simulink model "SimulinkElektrotechnikR2020"  (R2021b)
settings: Solver=FixedStepAuto  StartTime=0.0  StopTime=100  FixedStep=0.00001  RelTol=1e-3
undefined symbols (not defined in the file): C, L, R
settings Model: Creator=PM  LastModifiedBy=metzler
settings SolverCC: AlgebraicLoopSolver=TrustRegion
settings DebuggingCC: UnconnectedInputMsg=none  UnconnectedOutputMsg=none  UnconnectedLineMsg=none  SFMachineParentedDataDiag=warning
settings ModelReferenceCC: EnableRefExpFcnMdlSchedulingChecks=off

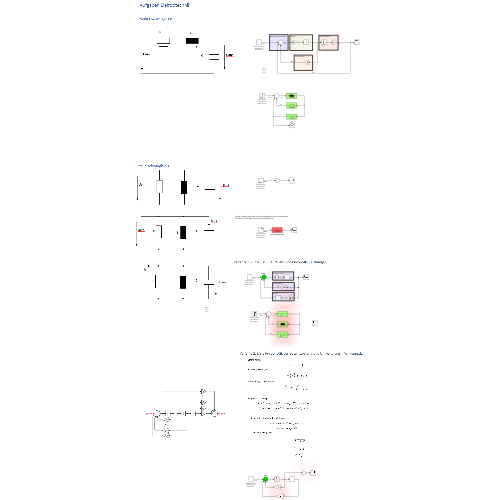
[thumbnail: Simulink's stored preview of the top-level diagram]
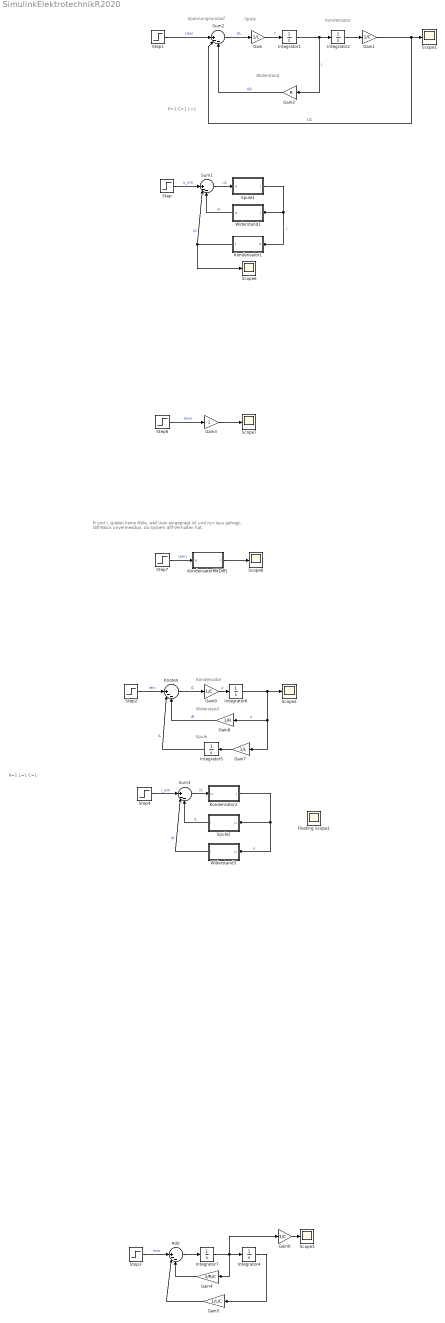
== system SimulinkElektrotechnikR2020 ==
  note: R und L  spielen keine Rolle, weil Uein eingeprägt ist und nur Iaus gefragt-
      | Diff-Block unvermeidbar, da System diff-Verhalten hat.
  note: R=1
      | L=1
      | C=1
  note: Widerstand
  note: Kondensator
  note: Spule
  note: Spannungsumlauf
  note: R=1
      | C=1
      | L=1
  note: Spule
  note: Widerstand
  note: Kondensator
  Add : Sum  Inputs=||+--
  Floating Scope1 : Scope
      settings: Floating=on
  Gain : Gain  Gain=1/L
  Gain1 : Gain  Gain=1/C
  Gain2 : Gain  Gain=R
  Gain3 : Gain
  Gain4 : Gain  Gain=1/R/C
  Gain5 : Gain  Gain=1/L/C
  Gain6 : Gain  Gain=1/C
  Gain7 : Gain  Gain=1/L
  Gain8 : Gain  Gain=1/R
  Gain9 : Gain  Gain=1/C
  Integrator{1..2,4..7} (6 alike) : Integrator
  Knoten : Sum  Inputs=||+--
  Kondensator1 : Subsystem  mask{C=1E-3}
      mask prompts: C "Kappazität C [F]"
      mask help:
      | Kapazität
      | Eingang ist u, Ausgang ist i.
      | i=1/C * integral(u)
      mask Display:
      | plot(0,0)
      | plot(100,100)
      | plot([0 0],[1 1]) %Umschalten auf dicke Linien
      | %patch([30 30 70 70 30],[40 60 60 40 40],[0,0,0])
      | plot([45 45],[40 60])
      | plot([55 55],[40 60])
      | plot([15 45],[50 50])
      | 
      | plot([55 85],[50 50])
      | 
      | 
      | 
      | text(30,19,['C=',num2str(C)])
      | 
      | 
      | 
      | port_label ('output',1,'u')
      | port_label ('input',1,'i')
  Kondensator2 : Subsystem  mask{C=C}
      mask prompts: C "Kappazität C [F]"
      mask help:
      | Kapazität
      | Eingang ist u, Ausgang ist i.
      | i=1/C * integral(u)
      mask Display:
      | plot(0,0)
      | plot(100,100)
      | plot([0 0],[1 1]) %Umschalten auf dicke Linien
      | %patch([30 30 70 70 30],[40 60 60 40 40],[0,0,0])
      | plot([45 45],[40 60])
      | plot([55 55],[40 60])
      | plot([15 45],[50 50])
      | 
      | plot([55 85],[50 50])
      | 
      | 
      | 
      | text(30,19,['C=',num2str(C)])
      | 
      | 
      | 
      | port_label ('output',1,'u')
      | port_label ('input',1,'i')
  KondensatorMitDiff1 : Subsystem  mask{C=1E-3}
      mask prompts: C "Kappazität C [F]"
      mask help:
      | Kapazität
      | Eingang ist u, Ausgang ist i.
      | i=C*u'
      | Wegen Diff-Block nicht für jeden Solver geeignet.
      mask Display:
      | plot(0,0)
      | plot(100,100)
      | plot([0 0],[1 1]) %Umschalten auf dicke Linien
      | %patch([30 30 70 70 30],[40 60 60 40 40],[0,0,0])
      | plot([45 45],[40 60])
      | plot([55 55],[40 60])
      | plot([15 45],[50 50])
      | 
      | plot([55 85],[50 50])
      | 
      | 
      | 
      | text(30,19,['C=',num2str(C)])
      | 
      | 
      | 
      | port_label ('output',1,'i')
      | port_label ('input',1,'u')
  Scope{1..3,6..8} (6 alike) : Scope
  Spule1 : Subsystem  mask{L=0.001}
      mask prompts: L "Induktivität L [H]"
      mask help:
      | Induktivität:
      | Eingang ist u, Ausgang ist i.
      mask Display:
      | plot(0,0)
      | plot(100,100)
      | plot([0 0],[1 1]) %Umschalten auf dicke Linien
      | patch([30 30 70 70 30],[35 65 65 35 35],[0,0,0])
      | plot([15 30],[50 50])
      | plot([70 88],[50 50])
      | text(30,20,['L=',num2str(L)])
      | port_label ('output',1,'i')
      | port_label ('input',1,'u')
  Spule2 : Subsystem  mask{L=L}
      mask prompts: L "Induktivität L [H]"
      mask help:
      | Induktivität:
      | Eingang ist u, Ausgang ist i.
      mask Display:
      | plot(0,0)
      | plot(100,100)
      | plot([0 0],[1 1]) %Umschalten auf dicke Linien
      | patch([30 30 70 70 30],[35 65 65 35 35],[0,0,0])
      | plot([15 30],[50 50])
      | plot([70 88],[50 50])
      | text(30,20,['L=',num2str(L)])
      | port_label ('output',1,'i')
      | port_label ('input',1,'u')
  Step{,1..4,6..7} (7 alike) : Step  SampleTime=0
      settings: AttributesFormatString=initial value=%<Before>\nfinal value=%<After>\nstep time=%<Time>
  Sum1 : Sum  Inputs=||+--
  Sum2 : Sum  Inputs=||+--
  Sum3 : Sum  Inputs=||+--
  Widerstand1 : Subsystem  mask{R=1000}
      mask prompts: R "Widerstand [Ohm]"
      mask help: Ohm'scher Widerstand, Eingang ist i, Ausgang ist u.
      mask Display:
      | plot(0,0)
      | plot(100,100)
      | plot([0 0],[1 1]) %Umschalten auf dicke Linien
      | plot([30 30 70 70 30],[35 65 65 35 35])
      | plot([15 30],[50 50])
      | plot([70 88],[50 50])
      | 
      | 
      | text(30,20,['R=',num2str(R)])
      | 
      | 
      | 
      | port_label ('output',1,'u')
      | port_label ('input',1,'i')
  Widerstand3 : Subsystem  mask{R=R}
      mask prompts: R "Widerstand [Ohm]"
      mask help: Ohm'scher Widerstand, Eingang ist u, Ausgang ist i.
      mask Display:
      | plot(0,0)
      | plot(100,100)
      | plot([0 0],[1 1]) %Umschalten auf dicke Linien
      | plot([30 30 70 70 30],[35 65 65 35 35])
      | plot([15 30],[50 50])
      | plot([70 88],[50 50])
      | 
      | 
      | text(30,20,['R=',num2str(R)])
      | 
      | 
      | 
      | port_label ('output',1,'i')
      | port_label ('input',1,'u')
  wires:
  Step1/1 -> Sum2/1  "Uein"
  Sum2/1 -> Gain/1  "UL"
  Gain/1 -> Integrator1/1  "I'"
  Integrator1/1 -> Gain2/1, Integrator2/1  "I"
  Integrator2/1 -> Gain1/1
  Gain1/1 -> Sum2/2, Scope1/1  "UC"
  Gain2/1 -> Sum2/3  "UR"
  Step2/1 -> Knoten/1  "Iein"
  Gain7/1 -> Integrator5/1
  Gain9/1 -> Integrator6/1  "u'"
  Knoten/1 -> Gain9/1  "iC"
  Gain8/1 -> Knoten/3  "iR"
  Integrator6/1 -> Scope2/1, Gain7/1, Gain8/1  "u"
  Integrator5/1 -> Knoten/2  "iL"
  Add/1 -> Integrator7/1
  Step3/1 -> Add/1  "Iein"
  Integrator7/1 -> Gain6/1, Gain4/1, Integrator4/1
  Gain4/1 -> Add/3
  Integrator4/1 -> Gain5/1
  Gain6/1 -> Scope3/1
  Step/1 -> Sum1/1  "u_ein"
  Widerstand1/1(u) -> Sum1/3  "ur"
  Kondensator1/1(i) -> Sum1/2, Scope6/1  "uc"
  Spule1/1(i) -> Kondensator1/1(u), Widerstand1/1(i)  "i"
  Sum1/1 -> Spule1/1(u)  "uL"
  Step6/1 -> Gain3/1  "Uein"
  Gain3/1 -> Scope7/1
  Step7/1 -> KondensatorMitDiff1/1(u)  "Uein"
  KondensatorMitDiff1/1(i) -> Scope8/1
  Sum3/1 -> Kondensator2/1(u)  "iC"
  Spule2/1(i) -> Sum3/3  "iL"
  Kondensator2/1(i) -> Widerstand3/1(u), Spule2/1(u)  "u"
  Widerstand3/1(i) -> Sum3/2  "iR"
  Step4/1 -> Sum3/1  "i_ein"
  Gain5/1 -> Add/2

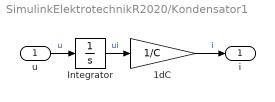
== system SimulinkElektrotechnikR2020/Kondensator1 ==
  u : Inport
  1dC : Gain  Gain=1/C
  Integrator : Integrator
  i : Outport  VectorParamsAs1DForOutWhenUnconnected=off
  wires:
  Integrator/1 -> 1dC/1  "ui"
  1dC/1 -> i/1  "i"
  u/1 -> Integrator/1  "u"

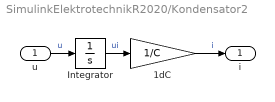
== system SimulinkElektrotechnikR2020/Kondensator2 ==
  u : Inport
  1dC : Gain  Gain=1/C
  Integrator : Integrator
  i : Outport  VectorParamsAs1DForOutWhenUnconnected=off
  wires:
  Integrator/1 -> 1dC/1  "ui"
  1dC/1 -> i/1  "i"
  u/1 -> Integrator/1  "u"

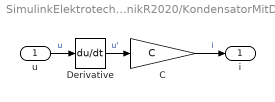
== system SimulinkElektrotechnikR2020/KondensatorMitDiff1 ==
  u : Inport
  C : Gain  Gain=C
  Derivative : Derivative
  i : Outport  VectorParamsAs1DForOutWhenUnconnected=off
  wires:
  Derivative/1 -> C/1  "u'"
  C/1 -> i/1  "i"
  u/1 -> Derivative/1  "u"

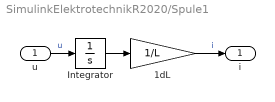
== system SimulinkElektrotechnikR2020/Spule1 ==
  u : Inport
  1dL : Gain  Gain=1/L
  Integrator : Integrator
  i : Outport  VectorParamsAs1DForOutWhenUnconnected=off
  wires:
  Integrator/1 -> 1dL/1
  1dL/1 -> i/1  "i"
  u/1 -> Integrator/1  "u"

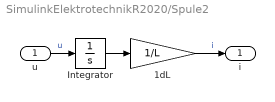
== system SimulinkElektrotechnikR2020/Spule2 ==
  u : Inport
  1dL : Gain  Gain=1/L
  Integrator : Integrator
  i : Outport  VectorParamsAs1DForOutWhenUnconnected=off
  wires:
  Integrator/1 -> 1dL/1
  1dL/1 -> i/1  "i"
  u/1 -> Integrator/1  "u"

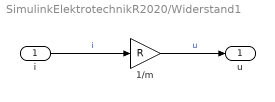
== system SimulinkElektrotechnikR2020/Widerstand1 ==
  i : Inport
  1/m : Gain  Gain=R
  u : Outport  VectorParamsAs1DForOutWhenUnconnected=off
  wires:
  1/m/1 -> u/1  "u"
  i/1 -> 1/m/1  "i"

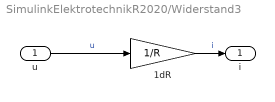
== system SimulinkElektrotechnikR2020/Widerstand3 ==
  u : Inport
  1dR : Gain  Gain=1/R
  i : Outport  VectorParamsAs1DForOutWhenUnconnected=off
  wires:
  1dR/1 -> i/1  "i"
  u/1 -> 1dR/1  "u"
